simulink model "mod_sim_VTMS"  (R2018b)
settings: Solver=FixedStepDiscrete  StartTime=0.0  StopTime=t_Simulation  FixedStep=delta_t  RelTol=1e-3
values from neighbouring files (symbols this model uses):
  P_charge = 150    [main_sim_VTMS.m]
undefined symbols (not defined in the file or in its folder): A_EMaschine_Getriebe, A_j_c, A_Stirn, Anzahl_Peltierelemente, b_Batteriepack, b_c, b_EMaschine, b_Getriebe, b_j, b_Ladegeraet, BatPara, c_W, delta_t, DiscIntNeverNeededParam, e_Fahrzeug, eta_EMaschine_Break_M_EMaschine, eta_EMaschine_Break_n_EMaschine, eta_EMaschine_Faktor_Volllast, eta_EMaschine_Table, eta_Getriebe, eta_Ladegeraet, eta_Leistungselektronik_Break_M_EMaschine, eta_Leistungselektronik_Break_n_EMaschine, eta_Leistungselektronik_Faktor_Volllast, eta_Leistungselektronik_Table, f_R, I_DT_U_Break_DT, I_DT_U_Break_U, I_DT_U_Value_I, i_Getriebe, I_max, Ladevorgang, M_EMaschine_max, m_Fahrzeug, m_Zuladung, n_Zelle, P_Nebenverbraucher, p_Zelle, Peltier_Max_Eff, Q_DT_U_Break_DT, Q_DT_U_Break_U, Q_DT_U_Value_Q, Q_Imax_DT_Break_DT, Q_Imax_DT_Value_Q, r_dynamisch, rho_Luft, s_Zelle, SOC_init, Steuerung_Kuehlerluefter, Steuerung_Pumpe, Steuerung_Ventil, switch_BP_Zyklus, T_Batteriepack_init, T_EMaschine_Getriebe_init, T_Ladegeraet_init, T_Ladegeraet_Offset, T_Leistungselektronik_init, T_Offset_Batteriepack, T_Offset_EMaschine_Getriebe, T_Offset_Leistungselektronik ... (+36)
libraries: simulink x3, simulink_extras x2
(part 5 of 5)

== system mod_sim_VTMS/Thermomanagementsystem/Batteriepack/Batteriepack(1) elektrisch/Zellmodell (abgeleitet aus Batteriepackmodell -> siehe FTM)/Potential der Zelle/ECM-Parameter Look-Ups ==
  T_Zelle [°C] : Inport
  I_Zelle [A] : Inport  Port=2
  BatState : Inport  Port=3
  Bus Creator : BusCreator  Inputs=7
  Bus Creator1 : BusCreator  Commented=on  Inputs=7
  Bus Selector : BusSelector  OutputSignals=SOC
  C1 : Lookup_n-D  Commented=on  BreakpointsForDimension1=BatPara.ECMPara.Dyn.EIS.SOCs  BreakpointsForDimension2=BatPara.ECMPara.Dyn.EIS.Temperatures  BeginIndexSearchUsingPreviousIndexResult=on  Table=BatPara.ECMPara.Dyn.EIS.C1  ExtrapMethod=Clip  UseLastTableValue=on  InternalRulePriority=Speed  RndMeth=Simplest  InputSameDT=on
  C2 : Lookup_n-D  Commented=on  BreakpointsForDimension1=BatPara.ECMPara.Dyn.EIS.SOCs  BreakpointsForDimension2=BatPara.ECMPara.Dyn.EIS.Temperatures  BeginIndexSearchUsingPreviousIndexResult=on  Table=BatPara.ECMPara.Dyn.EIS.C2  ExtrapMethod=Clip  UseLastTableValue=on  InternalRulePriority=Speed  RndMeth=Simplest  InputSameDT=on
  Constant : Constant  Value=BatPara.ECMPara.CN  VectorParams1D=off
  Divide : Product  Inputs=*/
  Lookup C1 : Lookup_n-D  NumberOfTableDimensions=3  BreakpointsForDimension1=BatPara.ECMPara.Dyn.Pulses.SOCs  BreakpointsForDimension2=BatPara.ECMPara.Dyn.Pulses.Temperatures  BreakpointsForDimension3=BatPara.ECMPara.Dyn.Pulses.C_rate  BeginIndexSearchUsingPreviousIndexResult=on  Table=BatPara.ECMPara.Dyn.Pulses.C1  ExtrapMethod=Clip  RemoveProtectionInput=on  UseLastTableValue=on  InternalRulePriority=Speed  RndMeth=Simplest  InputSameDT=on
  Lookup C2 : Lookup_n-D  NumberOfTableDimensions=3  BreakpointsForDimension1=BatPara.ECMPara.Dyn.Pulses.SOCs  BreakpointsForDimension2=BatPara.ECMPara.Dyn.Pulses.Temperatures  BreakpointsForDimension3=BatPara.ECMPara.Dyn.Pulses.C_rate  BeginIndexSearchUsingPreviousIndexResult=on  Table=BatPara.ECMPara.Dyn.Pulses.C2  ExtrapMethod=Clip  RemoveProtectionInput=on  UseLastTableValue=on  InternalRulePriority=Speed  RndMeth=Simplest  InputSameDT=on
  Lookup R1 : Lookup_n-D  NumberOfTableDimensions=3  BreakpointsForDimension1=BatPara.ECMPara.Dyn.Pulses.SOCs  BreakpointsForDimension2=BatPara.ECMPara.Dyn.Pulses.Temperatures  BreakpointsForDimension3=BatPara.ECMPara.Dyn.Pulses.C_rate  BeginIndexSearchUsingPreviousIndexResult=on  Table=BatPara.ECMPara.Dyn.Pulses.R1  ExtrapMethod=Clip  RemoveProtectionInput=on  UseLastTableValue=on  InternalRulePriority=Speed  RndMeth=Simplest  InputSameDT=on
  Lookup R2 : Lookup_n-D  NumberOfTableDimensions=3  BreakpointsForDimension1=BatPara.ECMPara.Dyn.Pulses.SOCs  BreakpointsForDimension2=BatPara.ECMPara.Dyn.Pulses.Temperatures  BreakpointsForDimension3=BatPara.ECMPara.Dyn.Pulses.C_rate  BeginIndexSearchUsingPreviousIndexResult=on  Table=BatPara.ECMPara.Dyn.Pulses.R2  ExtrapMethod=Clip  RemoveProtectionInput=on  UseLastTableValue=on  InternalRulePriority=Speed  RndMeth=Simplest  InputSameDT=on
  Lookup Ri : Lookup_n-D  NumberOfTableDimensions=3  BreakpointsForDimension1=BatPara.ECMPara.Dyn.Pulses.SOCs  BreakpointsForDimension2=BatPara.ECMPara.Dyn.Pulses.Temperatures  BreakpointsForDimension3=BatPara.ECMPara.Dyn.Pulses.C_rate  BeginIndexSearchUsingPreviousIndexResult=on  Table=BatPara.ECMPara.Dyn.Pulses.Ri  ExtrapMethod=Clip  RemoveProtectionInput=on  UseLastTableValue=on  InternalRulePriority=Speed  RndMeth=Simplest  InputSameDT=on
  R1 : Lookup_n-D  Commented=on  BreakpointsForDimension1=BatPara.ECMPara.Dyn.EIS.SOCs  BreakpointsForDimension2=BatPara.ECMPara.Dyn.EIS.Temperatures  BeginIndexSearchUsingPreviousIndexResult=on  Table=BatPara.ECMPara.Dyn.EIS.R1  ExtrapMethod=Clip  UseLastTableValue=on  InternalRulePriority=Speed  RndMeth=Simplest  InputSameDT=on
  R2 : Lookup_n-D  Commented=on  BreakpointsForDimension1=BatPara.ECMPara.Dyn.EIS.SOCs  BreakpointsForDimension2=BatPara.ECMPara.Dyn.EIS.Temperatures  BeginIndexSearchUsingPreviousIndexResult=on  Table=BatPara.ECMPara.Dyn.EIS.R2  ExtrapMethod=Clip  UseLastTableValue=on  InternalRulePriority=Speed  RndMeth=Simplest  InputSameDT=on
  Ri : Lookup_n-D  Commented=on  BreakpointsForDimension1=BatPara.ECMPara.Dyn.EIS.SOCs  BreakpointsForDimension2=BatPara.ECMPara.Dyn.EIS.Temperatures  BeginIndexSearchUsingPreviousIndexResult=on  Table=BatPara.ECMPara.Dyn.EIS.Rohm  ExtrapMethod=Clip  UseLastTableValue=on  InternalRulePriority=Speed  RndMeth=Simplest  InputSameDT=on
  T : Constant  Value=0.0001  VectorParams1D=off
  T1 : Constant  Commented=on  Value=0.0001  VectorParams1D=off
  BatPara_EIS : Outport
  BatPara_Pulses : Outport  Port=2
  wires:
  Bus Selector/1 -> Ri/1, R1/1, R2/1, C1/1, C2/1, Lookup C2/1, Lookup C1/1, Lookup R2/1, Lookup R1/1, Lookup Ri/1  "<SOC>"
  Divide/1 -> Lookup C2/2, Lookup C1/2, Lookup R2/2, Lookup R1/2, Lookup Ri/2
  Lookup Ri/1 -> Bus Creator/1  "R_i"
  T_Zelle [°C]/1 -> Ri/2, R1/2, R2/2, C1/2, C2/2, Lookup C1/3, Lookup Ri/3, Lookup R1/3, Lookup R2/3, Lookup C2/3  "T"
  Lookup R1/1 -> Bus Creator/2  "R_1"
  Lookup R2/1 -> Bus Creator/3  "R_2"
  Lookup C1/1 -> Bus Creator/4  "C_1"
  Lookup C2/1 -> Bus Creator/5  "C_2"
  BatState/1 -> Bus Selector/1
  R1/1 -> Bus Creator1/2  "R_1"
  C1/1 -> Bus Creator1/4  "C_1"
  R2/1 -> Bus Creator1/3  "R_2"
  C2/1 -> Bus Creator1/5  "C_2"
  I_Zelle [A]/1 -> Divide/1
  Constant/1 -> Bus Creator1/6, Divide/2, Bus Creator/6  "CN"
  Bus Creator/1 -> BatPara_Pulses/1
  Ri/1 -> Bus Creator1/1  "R_i"
  T/1 -> Bus Creator/7  "EnCo"
  T1/1 -> Bus Creator1/7  "EnCo"
  Bus Creator1/1 -> BatPara_EIS/1

== system mod_sim_VTMS/Thermomanagementsystem/Batteriepack/Batteriepack(1) elektrisch/Zellmodell (abgeleitet aus Batteriepackmodell -> siehe FTM)/Potential der Zelle/Hysteresespannung ==
  note: Zugrunde liegende Formel aus "Verbrugge, 2007 - Adaptive, multi-parameter battery state estimator with optimized time weighting factors"
  note: Wenn kein Hysteresemodell verwendet werden soll
      |  beta = 0 setzen
  BatState_In : Inport
  dt [s] : Inport  Port=2
  I_Zelle [A] : Inport  Port=3
  Add : Sum  Inputs=-+
  Add1 : Sum
  Bus Selector : BusSelector  OutputSignals=U_Hysterese,SOC
  Product : Product
  Product1 : Product  Inputs=4
  Sign : Signum
  V_H,max(SOC) : Lookup_n-D  NumberOfTableDimensions=1  BreakpointsForDimension1=BatPara.ECMPara.OCV.Steps.SOC_ch  BeginIndexSearchUsingPreviousIndexResult=on  Table=BatPara.ECMPara.OCV.Steps.U_hyst  ExtrapMethod=Clip  RemoveProtectionInput=on  UseLastTableValue=on  InternalRulePriority=Speed  RndMeth=Simplest  InputSameDT=on
  beta : Constant  Value=BatPara.ECMPara.OCV.Steps.beta_Hyst  VectorParams1D=off
  U_Hysterese [V] : Outport
  wires:
  I_Zelle [A]/1 -> Sign/1, Product1/3
  Bus Selector/2 -> V_H,max(SOC)/1  "<SOC>"
  V_H,max(SOC)/1 -> Add/2
  Add/1 -> Product1/4  "V_H,max-sign(I)*V_H"
  dt [s]/1 -> Product1/2
  Product1/1 -> Add1/2
  Add1/1 -> U_Hysterese [V]/1
  Sign/1 -> Product/2  "sign(I)"
  Product/1 -> Add/1
  BatState_In/1 -> Bus Selector/1
  Bus Selector/1 -> Add1/1, Product/1  "<U_Hysterese>"
  beta/1 -> Product1/1

== system mod_sim_VTMS/Thermomanagementsystem/Batteriepack/Batteriepack(1) elektrisch/Zellmodell (abgeleitet aus Batteriepackmodell -> siehe FTM)/Potential der Zelle/Ladezustandsabhängige Spannung ==
  SOC [-] : Inport
  BatPara : Inport  Port=2
  SOC --> U_SOC : Lookup_n-D  NumberOfTableDimensions=1  BreakpointsForDimension1=BatPara.ECMPara.OCV.Steps.SOC_ch  BreakpointsForDimension2=[1:3]  IndexSearchMethod=Linear search  BeginIndexSearchUsingPreviousIndexResult=on  Table=BatPara.ECMPara.OCV.Steps.U_mean  ExtrapMethod=Clip  RemoveProtectionInput=on  UseLastTableValue=on  RndMeth=Simplest  InputSameDT=on
  Terminator : Terminator
  U_SOC [V] : Outport
  wires:
  SOC [-]/1 -> SOC --> U_SOC/1
  SOC --> U_SOC/1 -> U_SOC [V]/1
  BatPara/1 -> Terminator/1

== system mod_sim_VTMS/Thermomanagementsystem/Batteriepack/Batteriepack(1) elektrisch/Zellmodell (abgeleitet aus Batteriepackmodell -> siehe FTM)/Potential der Zelle/SOC-Bestimmung ==
  note: Umrechnung Ah in As
  BatState_In : Inport
  BatPara : Inport  Port=2
  dt [s] : Inport  Port=3
  I_Zelle [A] : Inport  Port=4
  Bus Selector : BusSelector  OutputSignals=CN
  Bus Selector1 : BusSelector  OutputSignals=SOC
  Gain : Gain  Gain=3600
  Product : Product  Inputs=**/  RndMeth=Zero
  Sum : Sum
  SOC [-] : Outport
  wires:
  Bus Selector1/1 -> Sum/2  "<SOC>"
  Product/1 -> Sum/1  "dSOC"
  Bus Selector/1 -> Gain/1  "<CN>"
  Gain/1 -> Product/3
  I_Zelle [A]/1 -> Product/2
  dt [s]/1 -> Product/1
  BatState_In/1 -> Bus Selector1/1
  BatPara/1 -> Bus Selector/1
  Sum/1 -> SOC [-]/1

== system mod_sim_VTMS/Thermomanagementsystem/Batteriepack/Batteriepack(1) elektrisch/Zellmodell (abgeleitet aus Batteriepackmodell -> siehe FTM)/Potential der Zelle/Spannung am ersten RC-Glied ==
  BatState_In : Inport
  BatPara : Inport  Port=2
  dt [s] : Inport  Port=3
  I_Zelle [A] : Inport  Port=4
  Bus Selector : BusSelector  OutputSignals=U_RC1
  Bus Selector1 : BusSelector  OutputSignals=R_1,C_1
  Constant : Constant  VectorParams1D=off
  Gain : Gain  Gain=-1
  Math Function : Math  SaturateOnIntegerOverflow=on
  Product : Product  Inputs=**  RndMeth=Zero
  Product1 : Product  Inputs=/*  RndMeth=Zero
  Product2 : Product  Inputs=***  RndMeth=Zero
  Product3 : Product  Inputs=**  RndMeth=Zero
  Sum : Sum  Inputs=-+
  Sum1 : Sum
  U_RC1 [V] : Outport
  wires:
  Product/1 -> Product1/1
  Product3/1 -> Sum1/1
  Product1/1 -> Gain/1
  Sum1/1 -> U_RC1 [V]/1
  Gain/1 -> Math Function/1
  Product2/1 -> Sum1/2
  Bus Selector/1 -> Product3/1  "<U_RC1>"
  Math Function/1 -> Sum/1, Product3/2
  Sum/1 -> Product2/1
  Bus Selector1/1 -> Product2/2, Product/1  "<R_1>"
  BatPara/1 -> Bus Selector1/1
  dt [s]/1 -> Product1/2
  I_Zelle [A]/1 -> Product2/3
  BatState_In/1 -> Bus Selector/1
  Bus Selector1/2 -> Product/2  "<C_1>"
  Constant/1 -> Sum/2

== system mod_sim_VTMS/Thermomanagementsystem/Batteriepack/Batteriepack(1) elektrisch/Zellmodell (abgeleitet aus Batteriepackmodell -> siehe FTM)/Potential der Zelle/Spannung am zweiten RC-Glied ==
  BatState_In : Inport
  BatPara : Inport  Port=2
  dt [s] : Inport  Port=3
  I_Zelle [A] : Inport  Port=4
  Bus Selector : BusSelector  OutputSignals=U_RC2
  Bus Selector1 : BusSelector  OutputSignals=R_2,C_2
  Constant : Constant  VectorParams1D=off
  Gain : Gain  Gain=-1
  Math Function : Math  SaturateOnIntegerOverflow=on
  Product : Product  Inputs=**  RndMeth=Zero
  Product1 : Product  Inputs=/*  RndMeth=Zero
  Product2 : Product  Inputs=***  RndMeth=Zero
  Product3 : Product  Inputs=**  RndMeth=Zero
  Sum : Sum  Inputs=-+
  Sum1 : Sum
  U_RC2 [V] : Outport
  wires:
  BatPara/1 -> Bus Selector1/1
  BatState_In/1 -> Bus Selector/1
  Product/1 -> Product1/1
  Product3/1 -> Sum1/1
  Product1/1 -> Gain/1
  Gain/1 -> Math Function/1
  Product2/1 -> Sum1/2
  Math Function/1 -> Sum/1, Product3/2
  Sum/1 -> Product2/1
  dt [s]/1 -> Product1/2
  I_Zelle [A]/1 -> Product2/3
  Bus Selector/1 -> Product3/1  "<U_RC2>"
  Bus Selector1/2 -> Product/2  "<C_2>"
  Bus Selector1/1 -> Product2/2, Product/1  "<R_2>"
  Sum1/1 -> U_RC2 [V]/1
  Constant/1 -> Sum/2

== system mod_sim_VTMS/Thermomanagementsystem/Batteriepack/Batteriepack(1) elektrisch/Zellmodell (abgeleitet aus Batteriepackmodell -> siehe FTM)/Verlustleistung der Zelle/Irreversible Verlustleistung  ==
  note: Irreversible Verlustleistung der Zelle:
      |
      | -> basiert auf: P_Verlust_Zelle_irreversibel = R_Zelle_intern * I_Zelle^2
      |
      | -> R_Zelle_intern sind die internen Widerstände einer Zelle zu einem Auswertungszeitpunkt
  U_Ohm [V] : Inport
  U_RC1 [V] : Inport  Port=2
  U_RC2 [V] : Inport  Port=3
  I_Zelle [A] : Inport  Port=4
  Abs : Abs
  Add : Sum  Inputs=+++
  Product : Product  Inputs=**  RndMeth=Zero
  P_Verlust_Zelle_irreversibel [W] : Outport
  wires:
  I_Zelle [A]/1 -> Product/2
  Add/1 -> Product/1
  Product/1 -> Abs/1
  U_Ohm [V]/1 -> Add/1
  U_RC2 [V]/1 -> Add/3
  U_RC1 [V]/1 -> Add/2
  Abs/1 -> P_Verlust_Zelle_irreversibel [W]/1

== system mod_sim_VTMS/Thermomanagementsystem/Batteriepack/Batteriepack(1) elektrisch/Zellmodell (abgeleitet aus Batteriepackmodell -> siehe FTM)/Verlustleistung der Zelle/Reversible Verlustleistung ==
  note: R eversible Verlustleistung der Zelle:
      |
      | P_Verlust_Zelle_reversibel = - I_Zelle * T_Zelle * EnCo
      | = - I_Zelle * T_Zelle * (dU_OCV/dT_Cells)
      |
      | -> siehe bspw.: Eddahech et al., 2013 - Thermal characterization of a high-power lithium-ion battery
  I_Zelle [A] : Inport
  BatPara : Inport  Port=2
  T_Zelle [°C] : Inport  Port=3
  Bus Selector : BusSelector  OutputSignals=EnCo
  Gain : Gain  Gain=-1
  Product : Product  Inputs=***  RndMeth=Zero
  P_Verlust_Zelle_reversibel  [W] : Outport
  wires:
  Bus Selector/1 -> Product/2  "<EnCo>"
  Product/1 -> Gain/1
  BatPara/1 -> Bus Selector/1
  T_Zelle [°C]/1 -> Product/3
  I_Zelle [A]/1 -> Product/1
  Gain/1 -> P_Verlust_Zelle_reversibel  [W]/1

== matlab function mod_sim_VTMS/Thermomanagementsystem/Fluid/Fluid_Komponente thermisch/Energiestroeme 1. finites Volumen durch Kopplung mit vorheriger Fluid_Komponente - normal+Ventil/MATLAB Function ==
  data: u input; v input; a input; y output
function y = fcn(u,v,a)

n=size(u,1);
m=size(v,1);
y=zeros(n,1);
    
y(1,1)=a*(v(m,1)-u(1,1));

end

== matlab function mod_sim_VTMS/Thermomanagementsystem/Fluid/Fluid_Komponente thermisch/Energiestroeme 1. finites Volumen durch Kopplung mit vorherigen Fluid_Komponenten - Vereinigung/MATLAB Function ==
  data: u input; v input; w input; a input; y output; b input; c input; d input
function y = fcn(u,v,w,a,b,c,d)

n=size(u,1);
m=size(v,1);
l=size(w,1);
y=zeros(n,1);

y(1,1)=a*(c*v(m,1)+d*w(l,1)-b*u(1,1));

end

== matlab function mod_sim_VTMS/Thermomanagementsystem/Fluid/Fluid_Komponente thermisch/Energiestroeme finite Volumen innerhalb Fluid_Komponente/MATLAB Function ==
  data: u input; a input; y output
function y = fcn(u,a)

n=size(u,1);
y=zeros(n,1);

for i=2:n
    
    y(i,1)=a*(u(i-1,1)-u(i,1));

end
end

== matlab function mod_sim_VTMS/Thermomanagementsystem/Fluid/Fluid_Komponente thermisch/Konduktion 1. finites Volumen mit vorherigen Fluid_Komponenten - Vereinigung/MATLAB Function ==
  data: u input; y output; v input; w input; a input; b input
function y = fcn(u,v,w,a,b)

n=size(u,1);
m=size(v,1);
l=size(w,1);
y=zeros(n,1);

y(1,1)=(v(m,1)-u(1,1))/a+(w(l,1)-u(1,1))/b;                                 % Wärmeleistung für Fluidelement 1 durch Konduktion mit vorherigen Fluidelementen

end

== matlab function mod_sim_VTMS/Thermomanagementsystem/Fluid/Fluid_Komponente thermisch/Konduktion 1. finites Volumen mit vorheriger Fluid_Komponente - Ventil/MATLAB Function ==
  data: u input; y output; v input; a input
function y = fcn(u,v,a)

n=size(u,1);
m=size(v,1);
y=zeros(n,1);

y(1,1)=(v(m,1)-u(1,1))/a;                                                   % Wärmeleistung für Fluidelement 1 durch Konduktion mit vorherigen Fluidelement

end

== matlab function mod_sim_VTMS/Thermomanagementsystem/Fluid/Fluid_Komponente thermisch/Konduktion 1. finites Volumen mit vorheriger Fluid_Komponente - normal/MATLAB Function ==
  data: u input; y output; v input; a input
function y = fcn(u,v,a)

n=size(u,1);
m=size(v,1);
y=zeros(n,1);

y(1,1)=(v(m,1)-u(1,1))/a;                                                   % Wärmeleistung für Fluidelement 1 durch Konduktion mit vorherigen Fluidelement

end

== matlab function mod_sim_VTMS/Thermomanagementsystem/Fluid/Fluid_Komponente thermisch/Konduktion finite Volumen innerhalb Fluid_Komponente/MATLAB Function ==
  data: u input; y output; a input
function y = fcn(u,a)

n=size(u,1);
y=zeros(n,1);

for i=2:(n-1)
    
    y(i,1)=(u(i-1,1)+u(i+1,1)-2*u(i,1))/a;                                  % Wärmeleistung für Fluidelement i durch Konduktion mit vorherigen und nachkommenden Fluidelement

end

y(1,1)=(u(2,1)-u(1,1))/a;                                                   % Wärmeleistung für Fluidelement 1 durch Konduktion mit nachkommenden Fluidelement -> Konduktion mit vorherigen Fluidelement/en geht nur Kopplung mit anderen Temperaturvektor/en
y(n,1)=(u(n-1,1)-u(n,1))/a;                                                 % Wärmeleistung für Fluidelement n durch Konduktion mit vorherigen Fluidelement -> Konduktion mit nachkommenden Fluidelement/en geht nur Kopplung mit anderen Temperaturvektor/en


end

== matlab function mod_sim_VTMS/Thermomanagementsystem/Fluid/Fluid_Komponente thermisch/Konduktion n. finites Volumen mit nachfolgenden Fluid_Komponenten - Ventil/MATLAB Function ==
  data: u input; y output; v input; w input; a input; b input
function y = fcn(u,v,w,a,b)

n=size(u,1);
y=zeros(n,1);

y(n,1)=(v(1,1)-u(n,1))/a+(w(1,1)-u(n,1))/b;                                 % Wärmeleistung für Fluidelement n durch Konduktion mit nachkommenden Fluidelementen

end

== matlab function mod_sim_VTMS/Thermomanagementsystem/Fluid/Fluid_Komponente thermisch/Konduktion n. finites Volumen mit nachfolgender Fluid_Komponente - Vereinigung/MATLAB Function ==
  data: u input; y output; v input; a input
function y = fcn(u,v,a)

n=size(u,1);
y=zeros(n,1);

y(n,1)=(v(1,1)-u(n,1))/a;                                                   % Wärmeleistung für Fluidelement n durch Konduktion mit nachkommenden Fluidelement

end

== matlab function mod_sim_VTMS/Thermomanagementsystem/Fluid/Fluid_Komponente thermisch/Konduktion n. finites Volumen mit nachfolgender Fluid_Komponente - normal/MATLAB Function ==
  data: u input; y output; v input; a input
function y = fcn(u,v,a)

n=size(u,1);
y=zeros(n,1);

y(n,1)=(v(1,1)-u(n,1))/a;                                                   % Wärmeleistung für Fluidelement 1 durch Konduktion mit vorherigen Fluidelement

end
